simulink model "Lecture5Exercise"  (R2020b)
settings: Solver=VariableStepAuto  StartTime=0.0  StopTime=10.0  RelTol=1e-3
values from neighbouring files (symbols this model uses):
  A_aa = A_adj(1,1)    [Lecture5Exercises.m]
  A_ab = [A_adj(1,2) A_adj(1,3)]    [Lecture5Exercises.m]
  A_ba = [A_adj(2,1); A_adj(3,1)]    [Lecture5Exercises.m]
  A_bb = [A_adj(2,2) A_adj(2,3); A_adj(3,2) A_adj(3,3)]    [Lecture5Exercises.m]
  B_a = B_adj(1)    [Lecture5Exercises.m]
  B_b = [B_adj(2); B_adj(3)]    [Lecture5Exercises.m]
  C_adj = [Cd(3) Cd(2) Cd(1)]    [Lecture5Exercises.m]
  Gs = tf(10, [1 3 0])    [Assignment3.m]    (also in Lecture10_11Exercise.m = tf(num,den); Lecture3Exercise.m = tf(10, [1 2 0]); Lecture5Exercises.m = tf([4], [1 2 4 4]); Lecture6Exercise.m = tf(num,den))
  K = [KKi(1) KKi(2)]    [Lecture4Exercise.m]    (also in Lecture5Exercises.m = acker(A_adj, B_adj, [z_p z_p z_p]); Lecture9Exercise.m = P\D)
  L_er = acker(A_bb', A_ab', [z_per z_per])'    [Lecture5Exercises.m]
  Ts = 1.5    [Lecture3Exercise.m]    (also in Lecture4Exercise.m = 6; Lecture5Exercises.m = 0.02; Lecture6Exercise.m = 1/fs)
settings Model: Creator=sebastian  LastModifiedBy=sebastian

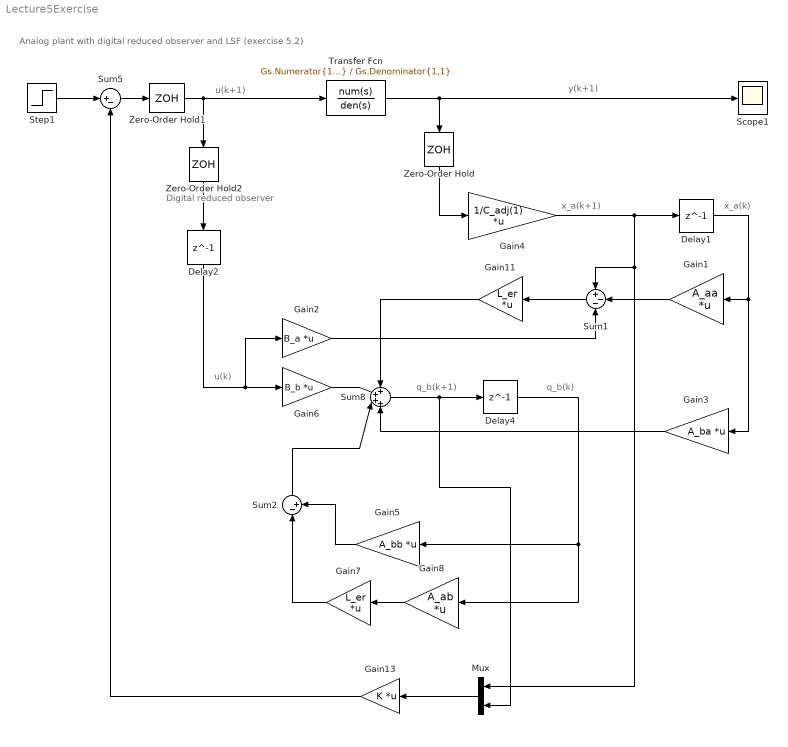
== system Lecture5Exercise ==
  note: u(k)
  note: Digital reduced observer
  note: x_a(k)
  note: x_a(k+1)
  note: y(k+1)
  note: u(k+1)
  note: q_b(k+1)
  note: Analog plant with digital reduced observer and LSF (exercise 5.2)
  note: q_b(k)
  Delay1 : Delay  DelayLength=1  InitialCondition=0  SampleTime=Ts
  Delay2 : Delay  DelayLength=1  InitialCondition=0  SampleTime=Ts
  Delay4 : Delay  DelayLength=1  InitialCondition=0  SampleTime=Ts
  Gain1 : Gain  Gain=A_aa  Multiplication=Matrix(K*u)
  Gain11 : Gain  Gain=L_er  Multiplication=Matrix(K*u)
  Gain13 : Gain  Gain=K  Multiplication=Matrix(K*u)
  Gain2 : Gain  Gain=B_a  Multiplication=Matrix(K*u)
  Gain3 : Gain  Gain=A_ba  Multiplication=Matrix(K*u)
  Gain4 : Gain  Gain=1/C_adj(1)  Multiplication=Matrix(K*u)
  Gain5 : Gain  Gain=A_bb  Multiplication=Matrix(K*u)
  Gain6 : Gain  Gain=B_b  Multiplication=Matrix(K*u)
  Gain7 : Gain  Gain=L_er  Multiplication=Matrix(K*u)
  Gain8 : Gain  Gain=A_ab  Multiplication=Matrix(K*u)
  Mux : Mux  Inputs=2
  Scope1 : Scope
  Step1 : Step  Time=0  SampleTime=0
  Sum1 : Sum  Inputs=+--
  Sum2 : Sum  Inputs=|-+
  Sum5 : Sum  Inputs=|+-
  Sum8 : Sum  Inputs=++++
  Transfer Fcn : TransferFcn  Numerator=Gs.Numerator{1,1}  Denominator=Gs.Denominator{1,1}
  Zero-Order Hold : ZeroOrderHold  SampleTime=Ts
  Zero-Order Hold1 : ZeroOrderHold  SampleTime=Ts
  Zero-Order Hold2 : ZeroOrderHold  SampleTime=Ts
  wires:
  Sum5/1 -> Zero-Order Hold1/1
  Delay4/1 -> Gain5/1, Gain8/1
  Gain11/1 -> Sum8/1
  Gain6/1 -> Sum8/2
  Sum8/1 -> Delay4/1, Mux/2
  Step1/1 -> Sum5/1
  Sum1/1 -> Gain11/1
  Delay1/1 -> Gain3/1, Gain1/1
  Gain1/1 -> Sum1/2
  Gain2/1 -> Sum1/3
  Gain3/1 -> Sum8/4
  Gain4/1 -> Mux/1, Sum1/1, Delay1/1
  Zero-Order Hold/1 -> Gain4/1
  Transfer Fcn/1 -> Scope1/1, Zero-Order Hold/1
  Gain13/1 -> Sum5/2
  Mux/1 -> Gain13/1
  Zero-Order Hold2/1 -> Delay2/1
  Delay2/1 -> Gain2/1, Gain6/1
  Sum2/1 -> Sum8/3
  Gain5/1 -> Sum2/2
  Gain8/1 -> Gain7/1
  Gain7/1 -> Sum2/1
  Zero-Order Hold1/1 -> Transfer Fcn/1, Zero-Order Hold2/1
